simulink library "Pipe"  (Simulink 8.2)
settings: Solver=ode45  StartTime=0.0  StopTime=10.0  RelTol=1e-3
libraries: carnot x4
settings Model: Creator=lena.frank  LastModifiedBy=drhf

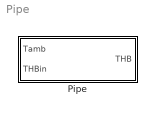
== system Pipe ==
  Pipe : Subsystem  mask(pipe){dia=0.02, len=10, hgt=5, uloss=100/20/10, cond=0, cwall=1000, t0=20, lin=100/0.2, qua=100/0.2^2, nodes=10}
      mask prompts: dia "diameter [m]"; len "length of pipe [m]"; hgt "static height [m], positive for outlet above"; uloss "heat losses per length [W/(m*K)]"; cond "effective conductivity in axial direction [W/(m*K)]"; cwall "capacity of pipewall per length in [J/(m*K)]"; t0 "initial temperature [degree Celsius]"; lin "pressure drop linear in massflow [Pa*s/kg]"; qua "pressure drop quadratic in massflow [Pa*s²/kg²]"; nodes "number of nodes"
      mask help:
      | Multinode pipe with capacity and simlified pressure drop calculation. The pressure drop is a quadratic function of the massflow. The dependance of the quadratic term on the Reynolds number is neglected. The flow is calculated by the upwind scheme heat conduction between nodes by central differences (Patankar 1980).
      | heat loss: ul = 2*Conductivity*pi*d_in*Length/Length/(d_in*ln(d_out/d_in))
      | The pressure change due to static height can usually be neglected for closes loop pumped systems.
      mask init:
      | if dia < 0.001
      |     dia = 0.001;
      |     disp('Warning in Pipe: diameter set to minimum value 0.001 m')
      | end
      | if len < 0.001
      |     len = 0.001;
      |     disp('Warning in Pipe: length set to minimum value 0.001 m')
      | end
      | if cwall < 0.001
      |     cwall = 0.001;
      |     disp('Warning in Pipe: heat capacity of the wall set to minimum value 0.001 m')
      | end
      | if nodes < 1
      |     nodes = 1;
      |     disp('Warning in Pipe: number of nodes set to minimum 1')
      | end
      mask Help: web(fullfile(path_carnot('help'),'Pipe.html'),'-helpbrowser')
      mask Display: plot(0,0,100,100,[24,27,27,24,75,80,80,75,24,20,20,24],[60,53,46,40,40,46,55,60,60,53,46,40])

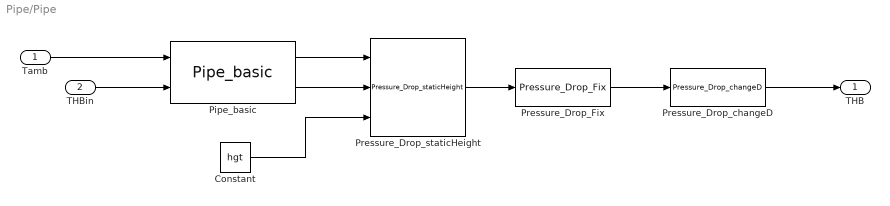
== system Pipe/Pipe ==
  Tamb : Inport
  THBin : Inport  Port=2
  Constant : Constant  Value=hgt
  Pipe_basic : carnot/Basic/Thermal_Models/Pipe_basic  vol=pi*(dia/2)^2*len  L=len  uloss=uloss  effcond=cond  cwall=cwall  t0=t0  nodes=nodes
  Pressure_Drop_Fix : carnot/Basic/Pressure_Drop/Pressure_Drop_Fix  con=0  lin=lin  qua=qua
  Pressure_Drop_changeD : carnot/Basic/Pressure_Drop/Pressure_Drop_changeD  dia=dia
  Pressure_Drop_staticHeight : carnot/Basic/Pressure_Drop/Pressure_Drop_staticHeight
  THB : Outport
  wires:
  Pressure_Drop_changeD/1 -> THB/1
  Pressure_Drop_Fix/1 -> Pressure_Drop_changeD/1
  Pressure_Drop_staticHeight/1 -> Pressure_Drop_Fix/1
  Constant/1 -> Pressure_Drop_staticHeight/3
  THBin/1 -> Pipe_basic/2
  Tamb/1 -> Pipe_basic/1
  Pipe_basic/1 -> Pressure_Drop_staticHeight/1
  Pipe_basic/2 -> Pressure_Drop_staticHeight/2
